simulink model "Stage10Abs"  (R2017b)
settings: Solver=ode15s  StartTime=0.  StopTime=150  MaxStep=0.1  RelTol=1e-8  AbsTol=1e-8  EnableMultiTasking=on
settings Model: ExtModeTrigMode=oneshot  ExtModeArmWhenConnect=off  Creator=LEVIENKL  LastModifiedBy=carlislt
settings DataIOCC: SaveFormat=Array  SignalLoggingSaveFormat=ModelDataLogs  SaveOutput=off  SaveTime=off  SignalLoggingName=sigsOut
settings OptimizationCC: BlockReduction=off  BooleanDataType=off  ExpressionDepthLimit=2147483647  InitFltsAndDblsToZero=on  LifeSpan=inf
settings DebuggingCC: SaveWithParameterizedLinksMsg=none  UnderspecifiedInitializationDetection=Classic  MergeDetectMultiDrivingBlocksExec=none  SignalResolutionControl=TryResolveAllWithWarning  MultiTaskDSMMsg=warning  MultiTaskCondExecSysMsg=none  FcnCallInpInsideContextMsg=warning  AllowSymbolicDim=off  StateNameClashWarn=warning  SFUnexpectedBacktrackingDiag=warning  SFNoUnconditionalDefaultTransitionDiag=warning  SFExecutionAtInitializationDiag=none
settings HardwareCC: ProdBitPerPointer=32  ProdBitPerSizeT=32  ProdBitPerPtrDiffT=32  ProdLargestAtomicFloat=None  ProdIntDivRoundTo=Undefined  ProdEndianess=Unspecified  ProdWordSize=32  ProdHWDeviceType=32-bit Generic  TargetUnknown=on
settings ModelReferenceCC: PropagateSignalLabelsOutOfModel=off
settings CodeAppCC: StateflowObjectComments=on
settings GRTTargetCC: TargetFcnLib=ansi_tfl_tmw.mat  TargetLangStandard=C89/C90 (ANSI)  GeneratePreprocessorConditionals=Disable all  CombineOutputUpdateFcns=off  GRTInterface=on
settings ConfigComp: CovMetricSettings=dw  CovHtmlReporting=on  CovSaveCumulativeToWorkspaceVar=on  CovSaveSingleToWorkspaceVar=on  CovExternalEMLEnable=off  CovSFcnEnable=off

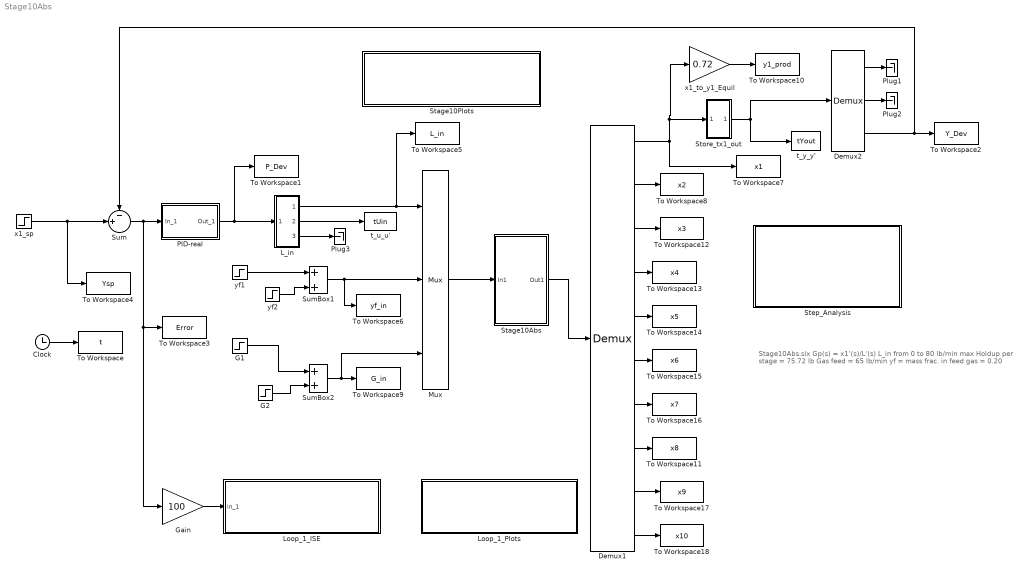
== system Stage10Abs ==
  note: Stage10Abs.slx
      | Gp(s) = x1'(s)/L'(s)
      | L_in from 0 to 80 lb/min max
      | Holdup per stage = 75.72 lb
      | Gas feed = 65 lb/min
      | yf = mass frac. in feed gas = 0.20
  Clock : Clock
  Demux1 : Demux  Outputs=10
  Demux2 : Demux  Outputs=3
  G1 : Step  Time=0  After=65  SampleTime=0
      settings: AttributesFormatString=%<Before> to %<After>\nat %<Time>
  G2 : Step  Time=5  After=0  SampleTime=0
      settings: AttributesFormatString=%<Before> to %<After>\nat %<Time>
  Gain : Gain  Gain=100  SaturateOnIntegerOverflow=on  OutDataTypeStr=Inherit: Same as input  ParamDataTypeStr=Inherit: Same as input
  L_in : Subsystem
  Loop_1_ISE : Subsystem  mask(Integral Squarred Evaluation - Loop 1){}
      settings: OpenFcn=ISE1
      mask Help: This block calculates and plots loop #1 ISE.
      mask Display: disp('After Loop 1 Simulation:\n Double Click for ISE evaluation\n (uses ISE1.p)')
  Loop_1_Plots : Subsystem  mask(Y,U,E Plots - Loop 1){}
      settings: OpenFcn=YPEplots
      mask Help: This block loop #1 Y,U,Error in 3x1 Figure Window.
      mask Display: disp('After Loop 1 Simulation:\n Double Click for Y, P, Error Plots\n (uses YPEplots.p)')
  Mux : Mux  Inputs=3
  PID-real : Subsystem  mask(PID(with alpha) Controller for ChE 461){Kc=-239, tauIi=1/14.9, tauD=0, alpha=0.05}
      mask prompts: Kc "Controller gain:"; tauIi "Inv of Integral time constant (careful - this is I action ! ) :"; tauD "Derivative time constant:"; alpha "Alpha value (small)::"
      mask help:
      | Enter expressions for controller gain,
      | inverse of integral time constant
      | and derivative time constant and alpha.
      settings: AttributesFormatString=Kc = %<Kc>\n1/TauI = %<tauIi>\nTauD = %<tauD>
      mask Help: This block implements a PID controller where parameters are entered for the Controller Gain, inverse of Integral time constant and Derivative time constant.  Alpha here is equal to 0.01.   Unmask this block to see how it works. The derivative term is implemented using a true derivative block.
      mask Display: disp('PIDalpha')
  Plug1 : Terminator
  Plug2 : Terminator
  Plug3 : Terminator
  Stage10Abs : Subsystem  mask(Absorber){xf=0, H=75.72, alpha=0.72, x1init=0.050000000000000, x2init=0.092509986698314, x3init=0.128651966080130, x4init=0.159379867335565, x5init=0.185504720808278, x6init=0.207716064280686, x7init=0.226600142591960, x8init=0.242655380948405, x9init=0.256305540327818, x10init=0.267910902200793}
      mask prompts: xf "Liq Feed mass frac."; H "StgHoldup"; alpha "Equil y=alpha*x"; x1init "Initial x1 mass frac. Btm Stage"; x2init "Initial x2 mass frac. Mid. Stage"; x3init "Initial x3 mass frac. Mid. Stage"; x4init "Initial x4 mass frac. Mid. Stage"; x5init "Initial x5 mass frac. Mid. Stage"; x6init "Initial x6 mass frac. Mid. Stage"; x7init "Initial x7 mass frac. Mid. Stage"; x8init "Initial x8 mass frac. Mid. Stage"; x9init "Initial x9 mass frac. Mid. Stage"; x10init "Initial x10 mass frac. Btm. Stage"
      mask help:
      | CHE 461 10-Stage Absorber
      | MATLAB v2015b
      | Dr. K.L. Levien
      | School of CBEE
      | Oregon State University
      | Corvallis, Oregon 97331-2702
      settings: AttributesFormatString=x1_0 = %<x1init>\n x2_0 = %<x2init>\n x3_0 = %<x3init>\n x4_0 = %<x4init>\n x5_0 = %<x5init>\n x6_0 = %<x6init>\n x7_0 = %<x7init>\n x8_0 = %<x8init>\n x9_0 = %<x9init>\n x10_0 = %<x10init>
      mask Help:
      | CHE 461 = Process Control
      | 10-stage Absorber, stage 1 = top, liq feed
      | See class handouts written by Dr. K.Levien
      | School of CBEE, Oregon State University
      mask Display: disp('Abs-10Stg')
  Stage10Plots : Subsystem  mask(Absorber Plots (10 stages)){}
      settings: OpenFcn=Stage10Plots
      mask Help: This block plots conditions from 10-stage absorber.
      mask Display: disp('After Absorber Simulation:\n Double Click for L,yf,G,x1,x10,y10 Plots\n (uses Stage10Plots.m)')
  Step_Analysis : Subsystem  mask(ASCII Datafile){}
      settings: OpenFcn=save tuin.dat tUin -ascii; save tyout.dat tYout -ascii; step2g
      mask Help: This block runs step2g\nin the MATLAB Command Window\nwith latest yout.dat data file.
      mask Display: disp('DOUBLE Click to\nRUN step2g\n\nGO TO Command Window !!')
  Store_tx1_out : Subsystem
  Sum : Sum  Inputs=-+|  SaturateOnIntegerOverflow=on  InputSameDT=on  OutDataTypeStr=Inherit: Same as first input
  SumBox1 : Sum
  SumBox2 : Sum
  To Workspace : ToWorkspace  VariableName=t  SampleTime=-1
  To Workspace1 : ToWorkspace  VariableName=P_Dev  SampleTime=-1
  To Workspace10 : ToWorkspace  VariableName=y1_prod  SampleTime=-1
  To Workspace11 : ToWorkspace  VariableName=x8  SampleTime=-1
  To Workspace12 : ToWorkspace  VariableName=x3  SampleTime=-1
  To Workspace13 : ToWorkspace  VariableName=x4  SampleTime=-1
  To Workspace14 : ToWorkspace  VariableName=x5  SampleTime=-1
  To Workspace15 : ToWorkspace  VariableName=x6  SampleTime=-1
  To Workspace16 : ToWorkspace  VariableName=x7  SampleTime=-1
  To Workspace17 : ToWorkspace  VariableName=x9  SampleTime=-1
  To Workspace18 : ToWorkspace  VariableName=x10  SampleTime=-1
  To Workspace2 : ToWorkspace  VariableName=Y_Dev  SampleTime=-1
  To Workspace3 : ToWorkspace  VariableName=Error  SampleTime=-1
  To Workspace4 : ToWorkspace  VariableName=Ysp  SampleTime=-1
  To Workspace5 : ToWorkspace  VariableName=L_in  SampleTime=-1
  To Workspace6 : ToWorkspace  VariableName=yf_in  SampleTime=-1
  To Workspace7 : ToWorkspace  VariableName=x1  SampleTime=-1
  To Workspace8 : ToWorkspace  VariableName=x2  SampleTime=-1
  To Workspace9 : ToWorkspace  VariableName=G_in  SampleTime=-1
  t_u_u' : ToWorkspace  VariableName=tUin
      settings: MaxDataPoints=3000
  t_y_y' : ToWorkspace  VariableName=tYout
      settings: MaxDataPoints=3000
  x1_sp : Step  Time=5  After=0  SampleTime=0
      settings: AttributesFormatString=%<Before> to %<After>\nat %<Time>
  x1_to_y1_Equil : Gain  Gain=0.72  SaturateOnIntegerOverflow=on  OutDataTypeStr=Inherit: Same as input  ParamDataTypeStr=Inherit: Same as input
  yf1 : Step  Time=0  After=0.2  SampleTime=0
      settings: AttributesFormatString=%<Before> to %<After>\nat %<Time>
  yf2 : Step  Time=5  After=0  SampleTime=0
      settings: AttributesFormatString=%<Before> to %<After>\nat %<Time>
  wires:
  Stage10Abs/1(Out1) -> Demux1/1
  Store_tx1_out/1(Outport) -> Demux2/1, t_y_y'/1
  Demux1/2 -> To Workspace8/1
  Mux/1 -> Stage10Abs/1(In1)
  L_in/1(out_1) -> Mux/1, To Workspace5/1
  x1_sp/1 -> To Workspace4/1, Sum/2
  Sum/1 -> PID-real/1(In_1), Gain/1, To Workspace3/1
  Demux2/1 -> Plug1/1
  Demux2/2 -> Plug2/1
  L_in/2(out_2) -> t_u_u'/1
  L_in/3(out_3) -> Plug3/1
  PID-real/1(Out_1) -> L_in/1(in_1), To Workspace1/1
  Gain/1 -> Loop_1_ISE/1(in_1)
  Clock/1 -> To Workspace/1
  Demux1/1 -> To Workspace7/1, Store_tx1_out/1(in_1), x1_to_y1_Equil/1
  Demux2/3 -> To Workspace2/1, Sum/1
  x1_to_y1_Equil/1 -> To Workspace10/1
  Demux1/3 -> To Workspace12/1
  Demux1/4 -> To Workspace13/1
  Demux1/5 -> To Workspace14/1
  Demux1/6 -> To Workspace15/1
  Demux1/7 -> To Workspace16/1
  yf1/1 -> SumBox1/1
  yf2/1 -> SumBox1/2
  SumBox1/1 -> To Workspace6/1, Mux/2
  SumBox2/1 -> Mux/3, To Workspace9/1
  G1/1 -> SumBox2/1
  G2/1 -> SumBox2/2
  Demux1/8 -> To Workspace11/1
  Demux1/9 -> To Workspace17/1
  Demux1/10 -> To Workspace18/1

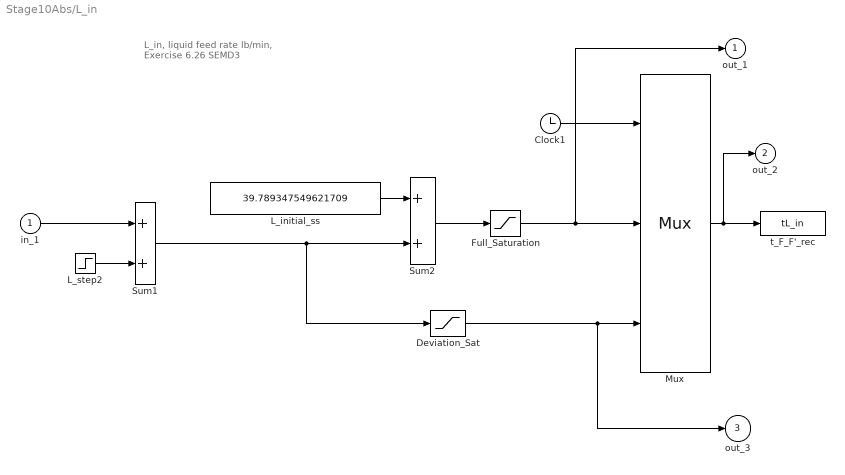
== system Stage10Abs/L_in ==
  note: L_in, liquid feed rate
      | lb/min, Exercise 6.26
      | SEMD3
  in_1 : Inport
  Clock1 : Clock
  Deviation_Sat : Saturate  UpperLimit=40.2106524503783  LowerLimit=-39.789347549621709  ZeroCross=off
      settings: AttributesFormatString=%<UpperLimit>\n%<LowerLimit>
  Full_Saturation : Saturate  UpperLimit=80  LowerLimit=0.001  ZeroCross=off
      settings: AttributesFormatString=%<UpperLimit>\n%<LowerLimit>
  L_initial_ss : Constant  Value=39.789347549621709
  L_step2 : Step  Time=5  After=0  SampleTime=0
      settings: AttributesFormatString=%<Before> to %<After>\nat %<Time>
  Mux : Mux  Inputs=3
  Sum1 : Sum  SaturateOnIntegerOverflow=on  InputSameDT=on  OutDataTypeStr=Inherit: Same as first input
  Sum2 : Sum  SaturateOnIntegerOverflow=on  InputSameDT=on  OutDataTypeStr=Inherit: Same as first input
  t_F_F'_rec : ToWorkspace  VariableName=tL_in
      settings: MaxDataPoints=3000
  out_1 : Outport
  out_2 : Outport  Port=2
  out_3 : Outport  Port=3
  wires:
  L_initial_ss/1 -> Sum2/1
  Clock1/1 -> Mux/1
  in_1/1 -> Sum1/1
  L_step2/1 -> Sum1/2
  Sum1/1 -> Deviation_Sat/1, Sum2/2
  Mux/1 -> t_F_F'_rec/1, out_2/1
  Sum2/1 -> Full_Saturation/1
  Full_Saturation/1 -> out_1/1, Mux/2
  Deviation_Sat/1 -> out_3/1, Mux/3

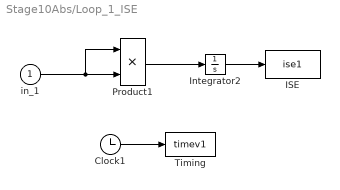
== system Stage10Abs/Loop_1_ISE ==
  in_1 : Inport
  Clock1 : Clock
  ISE : ToWorkspace  VariableName=ise1
      settings: MaxDataPoints=20000
  Integrator2 : Integrator
  Product1 : Product  SaturateOnIntegerOverflow=on  RndMeth=Zero  InputSameDT=on  OutDataTypeStr=Inherit: Same as first input
  Timing : ToWorkspace  VariableName=timev1
      settings: MaxDataPoints=20000
  wires:
  Product1/1 -> Integrator2/1
  Clock1/1 -> Timing/1
  Integrator2/1 -> ISE/1
  in_1/1 -> Product1/1, Product1/2

== system Stage10Abs/Loop_1_Plots ==

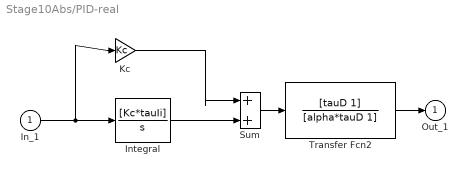
== system Stage10Abs/PID-real ==
  In_1 : Inport
  Integral : TransferFcn  Numerator=[Kc*tauIi]  Denominator=[1 0]
  Kc : Gain  Gain=Kc  SaturateOnIntegerOverflow=on  OutDataTypeStr=Inherit: Same as input  ParamDataTypeStr=Inherit: Same as input
  Sum : Sum  SaturateOnIntegerOverflow=on  InputSameDT=on  OutDataTypeStr=Inherit: Same as first input
  Transfer Fcn2 : TransferFcn  Numerator=[tauD 1]  Denominator=[alpha*tauD 1]
  Out_1 : Outport
  wires:
  Transfer Fcn2/1 -> Out_1/1
  Sum/1 -> Transfer Fcn2/1
  In_1/1 -> Integral/1, Kc/1
  Integral/1 -> Sum/2
  Kc/1 -> Sum/1

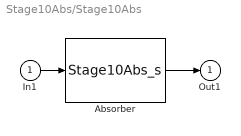
== system Stage10Abs/Stage10Abs ==
  In1 : Inport
  Absorber : S-Function  FunctionName=Stage10Abs_s  Parameters=xf,H,alpha,[x1init,x2init,x3init,x4init,x5init,x6init,x7init,x8init,x9init,x10init]  SFunctionDeploymentMode=off  EnableBusSupport=off
  Out1 : Outport
  wires:
  In1/1 -> Absorber/1
  Absorber/1 -> Out1/1

== system Stage10Abs/Stage10Plots ==

== system Stage10Abs/Step_Analysis ==

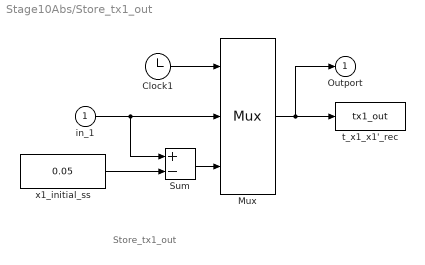
== system Stage10Abs/Store_tx1_out ==
  note: Store_tx1_out
  in_1 : Inport
  Clock1 : Clock
  Mux : Mux  Inputs=3
  Sum : Sum  Inputs=+-  SaturateOnIntegerOverflow=on  InputSameDT=on  OutDataTypeStr=Inherit: Same as first input
  t_x1_x1'_rec : ToWorkspace  VariableName=tx1_out
      settings: MaxDataPoints=3000
  x1_initial_ss : Constant  Value=0.05
  Outport : Outport
  wires:
  in_1/1 -> Mux/2, Sum/1
  x1_initial_ss/1 -> Sum/2
  Sum/1 -> Mux/3
  Clock1/1 -> Mux/1
  Mux/1 -> Outport/1, t_x1_x1'_rec/1
